simulink model "rejz"  (R2021a)
settings: Solver=VariableStepAuto  StartTime=0.0  StopTime=10.0  RelTol=1e-3
values from neighbouring files (symbols this model uses):
  R = conv(R1v, [1 -1])    [apr13.m]
  T = Bmv*Ao    [apr13.m]
  Ts = 0.2    [apr13.m]
libraries: cstblocks x3
settings Model: Creator=Peti  LastModifiedBy=Peti

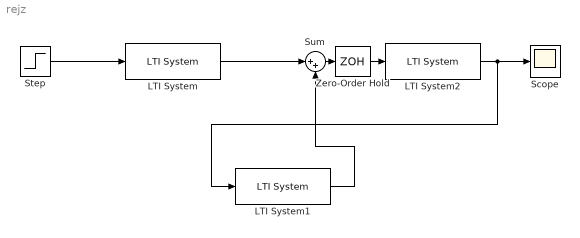
== system rejz ==
  LTI System : cstblocks/LTI System  sys=tf(T,R,Ts)  IC=[]
  LTI System1 : cstblocks/LTI System  sys=tf(1,[1 1])  IC=[]
  LTI System2 : cstblocks/LTI System  sys=tf(1,[1 1])  IC=[]
  Scope : Scope
  Step : Step  SampleTime=0
  Sum : Sum  Inputs=|++
  Zero-Order Hold : ZeroOrderHold  SampleTime=-1
  wires:
  LTI System/1 -> Sum/1
  LTI System2/1 -> LTI System1/1, Scope/1
  LTI System1/1 -> Sum/2
  Sum/1 -> Zero-Order Hold/1
  Zero-Order Hold/1 -> LTI System2/1
  Step/1 -> LTI System/1
